simulink subsystem "fifo25"  (R2022a)
settings: Solver=VariableStepAuto  StartTime=0.0  StopTime=10.0  RelTol=1e-3
undefined symbols (not defined in the file or in its folder): cols
libraries: simulink x5
settings Model: Creator=dileepan  LastModifiedBy=dileepan
settings DebuggingCC: UnconnectedInputMsg=warning  UnconnectedOutputMsg=warning  UnconnectedLineMsg=warning
settings RTWCC: DLArmComputeVersion=19.05

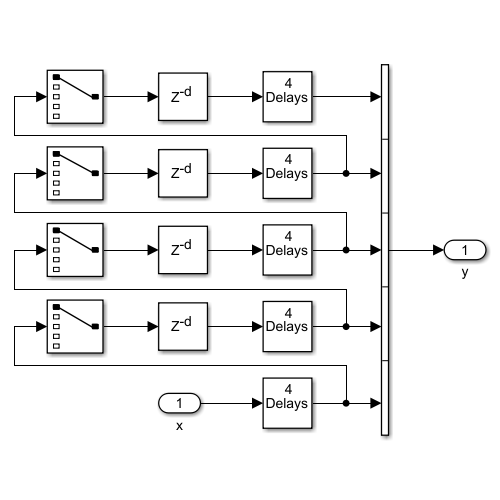
[thumbnail: Simulink's stored preview of the top-level diagram]
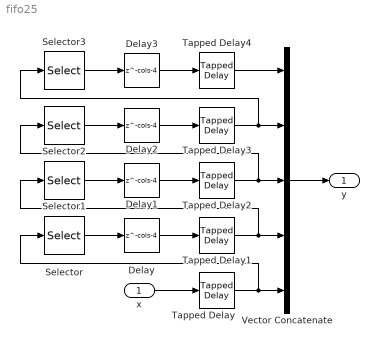
== system fifo25 ==
  x : Inport
  Delay{,1..3} (4 alike) : Delay  DelayLength=cols-4  UseCircularBuffer=on
  Selector{,1..3} (4 alike) : Selector  InputPortWidth=5  IndexOptions=Index vector (dialog)  Indices=1  OutputSizes=1
  Tapped Delay{,1..4} (5 alike) : simulink/Discrete/Tapped Delay  vinit=0.0  samptime=-1  NumDelays=4  DelayOrder=Oldest  includeCurrent=on
  Vector Concatenate : Concatenate  NumInputs=5
  y : Outport
  wires:
  Delay/1 -> Tapped Delay1/1
  x/1 -> Tapped Delay/1
  Delay1/1 -> Tapped Delay2/1
  Delay3/1 -> Tapped Delay4/1
  Delay2/1 -> Tapped Delay3/1
  Selector/1 -> Delay/1
  Selector1/1 -> Delay1/1
  Selector2/1 -> Delay2/1
  Selector3/1 -> Delay3/1
  Vector Concatenate/1 -> y/1
  Tapped Delay3/1 -> Vector Concatenate/2, Selector3/1
  Tapped Delay2/1 -> Vector Concatenate/3, Selector2/1
  Tapped Delay1/1 -> Vector Concatenate/4, Selector1/1
  Tapped Delay/1 -> Vector Concatenate/5, Selector/1
  Tapped Delay4/1 -> Vector Concatenate/1
